simulink model "model_DB"  (R2021b)
settings: Solver=VariableStepAuto  StartTime=0.0  StopTime=T  RelTol=1e-3
settings Model: Creator=mateusz  LastModifiedBy=mateusz

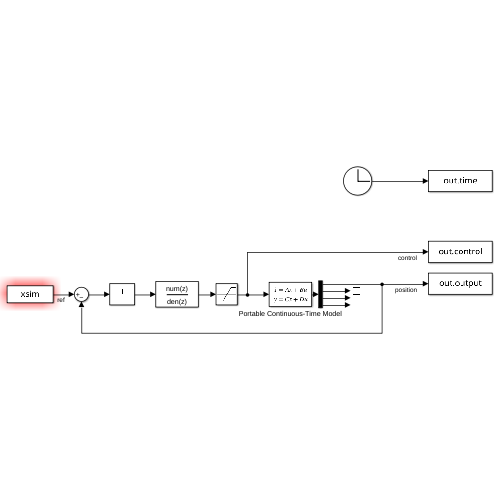
[thumbnail: Simulink's stored preview of the top-level diagram]
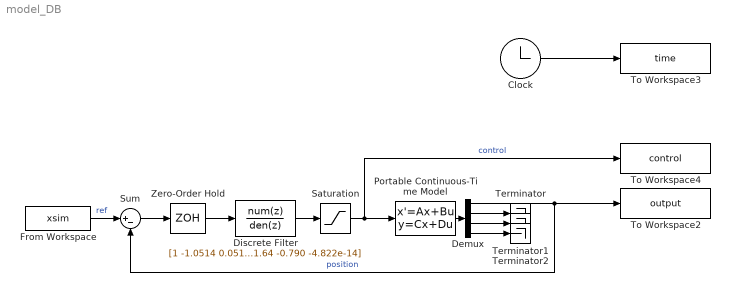
== system model_DB ==
  Clock : Clock
  Demux : Demux
  Discrete Filter : DiscreteFilter  Numerator=[1 -1.0514 0.0514 -2.331e-06 1.241e-26]  Denominator="[348.053 -215.626  -131.64 -0.790 -4.822e-14]"  SampleTime=2
  From Workspace : FromWorkspace  VariableName=xsim
  Portable Continuous-Time Model : StateSpace  A=|  B=[0;0;0;2.59e4];  C=eye(4,4)  D=zeros(4,1)  InitialCondition=0
      | [0  1  0    0;
      |      0 -5  4.5  0;
      |      0  0 -0.7108*2  23.6012*2;
      |      0  0 -5.3898 -4040];
  Saturation : Saturate
  Sum : Sum  Inputs=|+-
  Terminator : Terminator
  Terminator1 : Terminator
  Terminator2 : Terminator
  To Workspace2 : ToWorkspace  VariableName=output  SampleTime=0.02
  To Workspace3 : ToWorkspace  VariableName=time  SampleTime=0.02
  To Workspace4 : ToWorkspace  VariableName=control  SampleTime=0.02
  Zero-Order Hold : ZeroOrderHold  SampleTime=2
  wires:
  Portable Continuous-Time Model/1 -> Demux/1
  Demux/3 -> Terminator1/1
  Demux/4 -> Terminator2/1
  Clock/1 -> To Workspace3/1
  Demux/2 -> Terminator/1
  Demux/1 -> To Workspace2/1, Sum/2  "position"
  From Workspace/1 -> Sum/1  "ref"
  Saturation/1 -> To Workspace4/1, Portable Continuous-Time Model/1  "control"
  Sum/1 -> Zero-Order Hold/1
  Discrete Filter/1 -> Saturation/1
  Zero-Order Hold/1 -> Discrete Filter/1
